simulink model "dft_ex10_1"  (R2016b)
settings: Solver=VariableStepAuto  StartTime=0.0  StopTime=10.0  RelTol=1e-3
libraries: dspxfrm3 x2
settings Model: Creator=eechris  LastModifiedBy=eechris

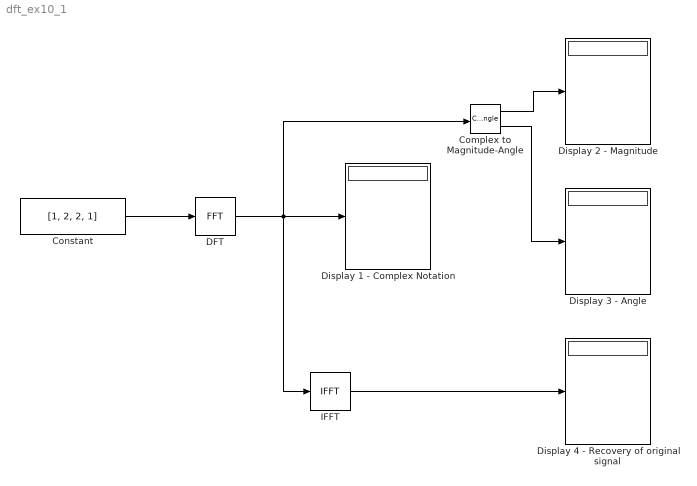
== system dft_ex10_1 ==
  Complex to Magnitude-Angle : ComplexToMagnitudeAngle
  Constant : Constant  Value=[1, 2, 2, 1]
  DFT : dspxfrm3/FFT  FFTImplementation=Auto  CompMethod=Table lookup  TableOpt=NEW  TableOptActive=Speed  BitRevOrder=off  Normalize=off  InheritFFTLength=on  FFTLength=64  WrapInput=on  roundingMode=Floor  overflowMode=off  firstCoeffDataTypeStr=Inherit: Same word length as input  firstCoeffLastDataTypeStr=Inherit: Same word length as input  outputMin=[]  outputMax=[]
  Display 1 - Complex Notation : Display
  Display 2 - Magnitude : Display
  Display 3 - Angle : Display
  Display 4 - Recovery of original signal : Display
  IFFT : dspxfrm3/IFFT  FFTImplementation=Auto  CompMethod=Table lookup  TableOpt=NEW  TableOptActive=Speed  BitRevOrder=off  cs_in=off  Normalize=on  InheritFFTLength=on  FFTLength=64  WrapInput=on  mode=Complex  outSamplingMode=Sample based  roundingMode=Floor  overflowMode=off  firstCoeffDataTypeStr=Inherit: Same word length as input  firstCoeffLastDataTypeStr=Inherit: Same word length as input  outputMin=[]  outputMax=[]
  wires:
  Constant/1 -> DFT/1
  DFT/1 -> IFFT/1, Complex to Magnitude-Angle/1, Display 1 - Complex Notation/1
  Complex to Magnitude-Angle/1 -> Display 2 - Magnitude/1
  Complex to Magnitude-Angle/2 -> Display 3 - Angle/1
  IFFT/1 -> Display 4 - Recovery of original signal/1
